simulink model "SPWM_Three_Phase_Inverter"  (R2025a)
settings: Solver=ode23tb  StartTime=0.0  StopTime=0.3  MaxStep=1e-4  RelTol=1e-3
libraries: spsIGBTDiodeLib x6, spsSeriesRLCBranchLib x3, spsSawtoothGeneratorLib x3, spsGroundLib x1, spsThreePhaseVIMeasurementLib x1, spsDCVoltageSourceLib x1, sps_lib x1
settings Model: Creator=Jawad  LastModifiedBy=Jawad

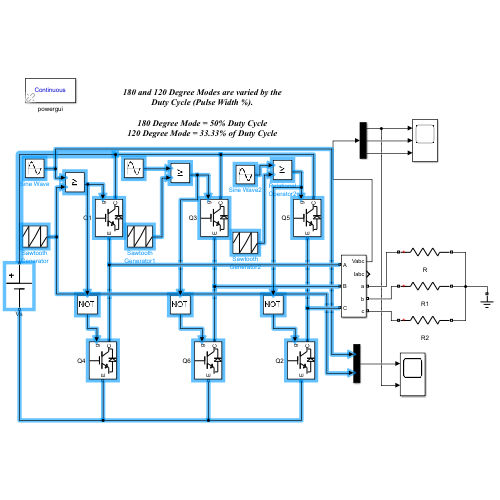
[thumbnail: Simulink's stored preview of the top-level diagram]
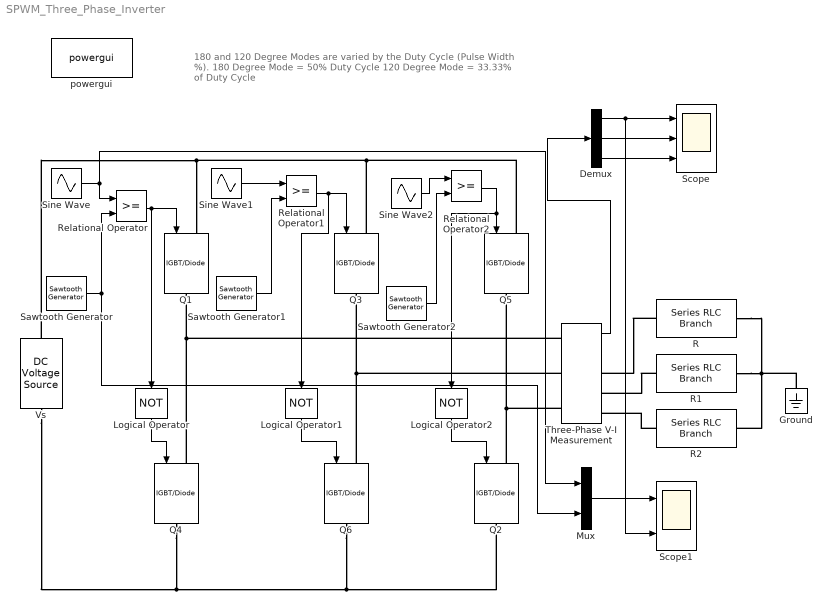
== system SPWM_Three_Phase_Inverter ==
  note: 180 and 120 Degree Modes are varied by the Duty Cycle (Pulse Width %).
      |
      | 180 Degree Mode = 50% Duty Cycle
      | 120 Degree Mode = 33.33% of Duty Cycle
  Demux : Demux  Outputs=3
  Ground : spsGroundLib/Ground  LConnTagsString=a
  Logical Operator : Logic  Operator=NOT  AllPortsSameDT=off  OutDataTypeStr=boolean
  Logical Operator1 : Logic  Operator=NOT  AllPortsSameDT=off  OutDataTypeStr=boolean
  Logical Operator2 : Logic  Operator=NOT  AllPortsSameDT=off  OutDataTypeStr=boolean
  Mux : Mux  Inputs=2
  Q{1..6} (6 alike) : spsIGBTDiodeLib/IGBT//Diode  Ron=1e-3  Rs=1e5  Cs=inf  Measurements=off
  R : spsSeriesRLCBranchLib/Series RLC Branch  LConnTagsString=__new0  RConnTagsString=__new0  BranchType=R  Resistance=10  Inductance=1e-3  SetiL0=off  InitialCurrent=0  Capacitance=1e-6  Setx0=off  InitialVoltage=0  Measurements=None
  R1 : spsSeriesRLCBranchLib/Series RLC Branch  LConnTagsString=__new0  RConnTagsString=__new0  BranchType=R  Resistance=10  Inductance=1e-3  SetiL0=off  InitialCurrent=0  Capacitance=1e-6  Setx0=off  InitialVoltage=0  Measurements=None
  R2 : spsSeriesRLCBranchLib/Series RLC Branch  LConnTagsString=__new0  RConnTagsString=__new0  BranchType=R  Resistance=10  Inductance=1e-3  SetiL0=off  InitialCurrent=0  Capacitance=1e-6  Setx0=off  InitialVoltage=0  Measurements=None
  Relational Operator : RelationalOperator  OutDataTypeStr=boolean  RndMeth=Simplest  InputSameDT=off
  Relational Operator1 : RelationalOperator  OutDataTypeStr=boolean  RndMeth=Simplest  InputSameDT=off
  Relational Operator2 : RelationalOperator  OutDataTypeStr=boolean  RndMeth=Simplest  InputSameDT=off
  Sawtooth Generator : spsSawtoothGeneratorLib/Sawtooth Generator  Freq=1000  Phase=180  Ts=0
  Sawtooth Generator1 : spsSawtoothGeneratorLib/Sawtooth Generator  Freq=1000  Phase=180  Ts=0
  Sawtooth Generator2 : spsSawtoothGeneratorLib/Sawtooth Generator  Freq=1000  Phase=180  Ts=0
  Scope : Scope  NumInputPorts=3
      settings: ActiveDisplayString=3  Title=Vc  ActiveDisplayYMinimum=-83.324999166916641  ActiveDisplayYMaximum=83.324999166916641
  Scope1 : Scope  NumInputPorts=2
      settings: Title=Va  ActiveDisplayYMinimum=-83.324999166916655  ActiveDisplayYMaximum=83.324999166916683
  Sine Wave : Sin  Amplitude=0.9  Frequency=2*pi*50  SampleTime=0
  Sine Wave1 : Sin  Amplitude=0.9  Frequency=2*pi*50  Phase=120*(pi/180)  SampleTime=0
  Sine Wave2 : Sin  Amplitude=0.9  Frequency=2*pi*50  Phase=240*(pi/180)  SampleTime=0
  Three-Phase V-I Measurement : spsThreePhaseVIMeasurementLib/Three-Phase V-I Measurement  VoltageMeasurement=phase-to-ground  SetLabelV=off  LabelV=Vabc  Vpu=off  VpuLL=off  CurrentMeasurement=yes  SetLabelI=off  LabelI=Iabc  Ipu=off  Pbase=100e6  Vbase=500e3  OutputType=Complex  PhasorSimulation=off  PSBequivalent=0
  Vs : spsDCVoltageSourceLib/DC Voltage Source  Amplitude=100  Measurements=None
  powergui : sps_lib/powergui  Priority=1  SimulationMode=Continuous  SampleTime=50e-6  frequency=60  Iterations=50  frequencyindice=0  Pbase=100e6  ErrMax=1e-4  UnitsV=kV  UnitsW=MW  buscounter=0  FunctionMessages=off  echomessages=off  EnableUseOfTLC=off  CurrentSourceSwitches=off  DisableSnubberDevices=off  DisableRonSwitches=off  DisableVfSwitches=off  DisplayEquations=off  AutomaticDiscreteSolvers=off  SolverType=Tustin/Backward Euler (TBE)  Interpol=off  ExternalGateDelay=off  methode=off  Ts=100  x0status=blocks  SPID=on  SwTol=0  HookPort=off  NonlinearTolerance=1e-4  nMaxIteration=100  ContinueOnMaxIteration=off  RestoreLinks=warning  ResistiveCurrentMeasurement=off  Frange=[0:2:500]  Ylog=off  Xlog=on  ShowGrid=off  save=off  variable=ZData  structure=0  ZoomFFT=off  StartTime=0.0  cycles=1  DisplayStyle=1  fundamental=60  FreqAxis=off  MaxFrequency=1000  frequencyindicesteady=1  RmsSteady=1  display=off
  wires:
  Demux/2 -> Scope/2
  Demux/1 -> Scope1/2, Scope/1
  Demux/3 -> Scope/3
  Three-Phase V-I Measurement/1 -> Demux/1
  Sine Wave/1 -> Mux/1, Relational Operator/1
  Sine Wave1/1 -> Relational Operator1/1
  Sawtooth Generator1/1 -> Relational Operator1/2
  Relational Operator1/1 -> Logical Operator1/1, Q3/1
  Sawtooth Generator2/1 -> Relational Operator2/2
  Sine Wave2/1 -> Relational Operator2/1
  Relational Operator2/1 -> Logical Operator2/1, Q5/1
  Relational Operator/1 -> Q1/1, Logical Operator/1
  Logical Operator/1 -> Q4/1
  Logical Operator1/1 -> Q6/1
  Logical Operator2/1 -> Q2/1
  Mux/1 -> Scope1/1
  Sawtooth Generator/1 -> Mux/2, Relational Operator/2
  connections:
  Q2/RConn1 -- Q4/RConn1 -- Vs/LConn1 -- Q6/RConn1
  Q5/LConn1 -- Q3/LConn1 -- Vs/RConn1 -- Q1/LConn1
  R/RConn1 -- Ground/LConn1 -- R1/RConn1 -- R2/RConn1
  Q3/RConn1 -- Q6/LConn1 -- Three-Phase V-I Measurement/LConn2
  Q1/RConn1 -- Three-Phase V-I Measurement/LConn1 -- Q4/LConn1
  Q5/RConn1 -- Q2/LConn1 -- Three-Phase V-I Measurement/LConn3
  R1/LConn1 -- Three-Phase V-I Measurement/RConn2
  R/LConn1 -- Three-Phase V-I Measurement/RConn1
  R2/LConn1 -- Three-Phase V-I Measurement/RConn3
